simulink model "LQ_integrator_kalman_pendulum_anim"  (Simulink 8.8)
settings: Solver=ode45  StartTime=0.0  StopTime=inf  RelTol=1e-3  EnableMultiTasking=on
values from neighbouring files (symbols this model uses):
  A_kalman = A - L*C    [pendulum_sys_init_solution.m]
  B_kalman = [L B-L*D]    [pendulum_sys_init_solution.m]
  C_kalman = eye(4)    [pendulum_sys_init_solution.m]
  D_kalman = zeros(4,3)    [pendulum_sys_init_solution.m]
  g = 9.81    [pendulum_sys_init_solution.m]
  K_LQ = lqr(A_int,B_int,Q,R)    [pendulum_sys_init_solution.m]
  kc = 2    [pendulum_sys_init_solution.m]
  ke = 2    [pendulum_sys_init_solution.m]
  l = 1    [pendulum_sys_init_solution.m]
  M = 10    [pendulum_sys_init_solution.m]
  m = 2    [pendulum_sys_init_solution.m]
  ra = 10    [pendulum_sys_init_solution.m]
  rr = .1    (= 0.1)    [pendulum_sys_init_solution.m]
undefined symbols (not defined in the file or in its folder): pendolo_sys_diff
libraries: simulink x1, vrlib x1
settings Model: Creator=Titano  LastModifiedBy=AlessioLaBella
settings OptimizationCC: ExpressionDepthLimit=2147483647  InitFltsAndDblsToZero=on
settings DebuggingCC: SolverPrmCheckMsg=warning
settings SimMechanicsCC: VisDuringSimulation=on
settings ConfigurationSet: Description=SimMechanics 2G

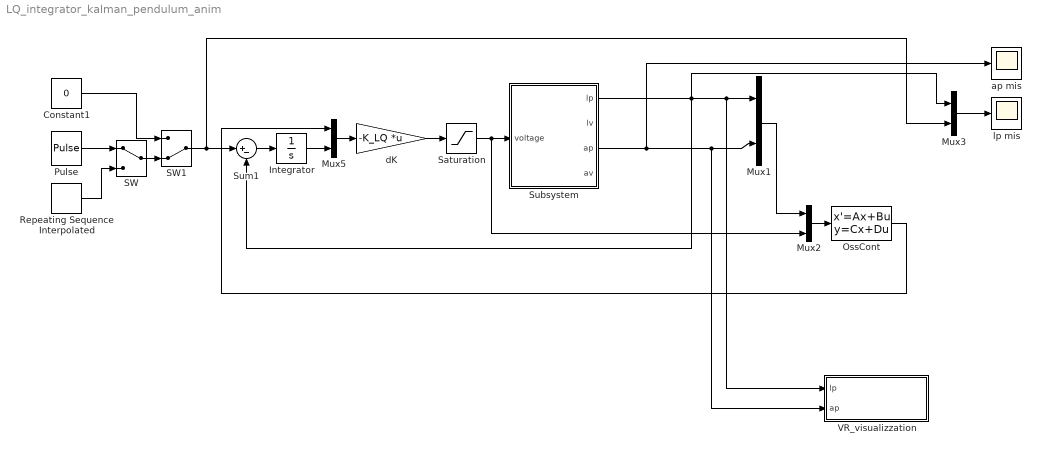
== system LQ_integrator_kalman_pendulum_anim ==
  Constant1 : Constant  Value=0
  Integrator : Integrator
  Mux{1..3,5} (4 alike) : Mux  Inputs=2
  OssCont : StateSpace  A=A_kalman  B=B_kalman  C=C_kalman  D=D_kalman  X0=0
  Pulse : DiscretePulseGenerator  PulseType=Time based  Amplitude=.5  Period=20  PulseWidth=50
  Repeating Sequence Interpolated : simulink/Sources/Repeating Sequence Interpolated  OutValues=[.5 -.5 -.5 .5 .5].'  TimeValues=[0 2.5 5 7.5 10].'  LookUpMeth=Interpolation-Use End Values  tsamp=0.01  OutMin=[]  OutMax=[]  OutDataTypeStr=float('double')  OutputDataTypeScalingMode=Specify via dialog  OutDataType=float('double')  OutScaling=2^-10
  SW : ManualSwitch
  SW1 : ManualSwitch  CurrentSetting=0
  Saturation : Saturate  UpperLimit=24  LowerLimit=-24
  Subsystem : Subsystem
  Sum1 : Sum  Inputs=|+-
  VR_visualizzation : Subsystem
  ap mis : Scope
  dK : Gain  Gain=-K_LQ  Multiplication=Matrix(K*u)
  lp mis : Scope
  wires:
  Mux2/1 -> OssCont/1
  Subsystem/3(ap) -> ap mis/1, Mux1/2, VR_visualizzation/2(ap)
  Subsystem/1(lp) -> Mux3/1, Sum1/2, Mux1/1, VR_visualizzation/1(lp)
  Mux3/1 -> lp mis/1
  Constant1/1 -> SW1/1
  OssCont/1 -> Mux5/1
  SW1/1 -> Mux3/2, Sum1/1
  Sum1/1 -> Integrator/1
  Integrator/1 -> Mux5/2
  dK/1 -> Saturation/1
  Mux5/1 -> dK/1
  Saturation/1 -> Mux2/2, Subsystem/1(voltage)
  SW/1 -> SW1/2
  Pulse/1 -> SW/1
  Repeating Sequence Interpolated/1 -> SW/2
  Mux1/1 -> Mux2/1

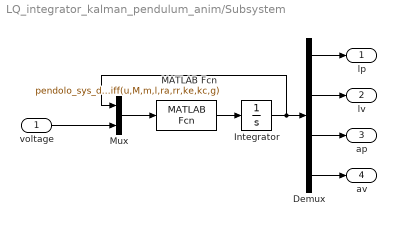
== system LQ_integrator_kalman_pendulum_anim/Subsystem ==
  voltage : Inport
  Demux : Demux
  Integrator : Integrator  InitialCondition=[0 0 0 0]
  MATLAB Fcn : MATLABFcn  MATLABFcn=pendolo_sys_diff(u,M,m,l,ra,rr,ke,kc,g)
  Mux : Mux  Inputs=2
  lp : Outport
  lv : Outport  Port=2
  ap : Outport  Port=3
  av : Outport  Port=4
  wires:
  MATLAB Fcn/1 -> Integrator/1
  Integrator/1 -> Demux/1, Mux/1
  Demux/4 -> av/1
  Demux/3 -> ap/1
  Demux/2 -> lv/1
  Demux/1 -> lp/1
  Mux/1 -> MATLAB Fcn/1
  voltage/1 -> Mux/2

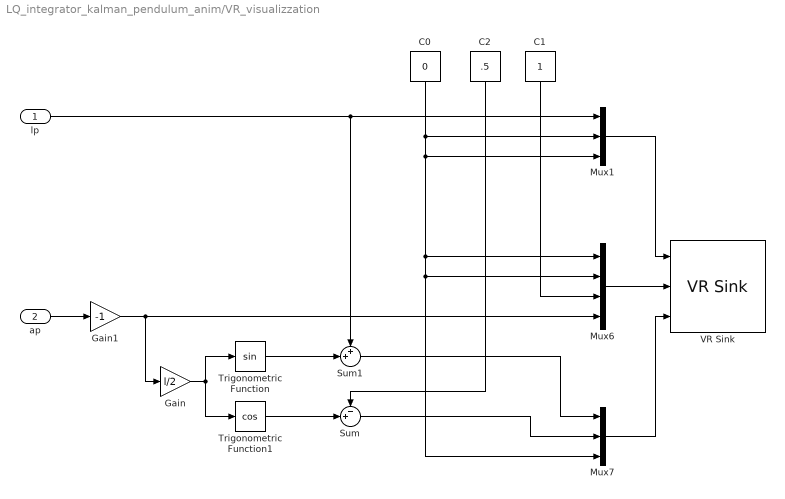
== system LQ_integrator_kalman_pendulum_anim/VR_visualizzation ==
  lp : Inport
  ap : Inport  Port=2
  C0 : Constant  Value=0
  C1 : Constant
  C2 : Constant  Value=.5
  Gain : Gain  Gain=l/2
  Gain1 : Gain  Gain=-1
  Mux1 : Mux  Inputs=3
  Mux6 : Mux
  Mux7 : Mux  Inputs=3
  Sum : Sum  Inputs=-+|
  Sum1 : Sum  Inputs=++|
  Trigonometric Function : Trigonometry
  Trigonometric Function1 : Trigonometry  Operator=cos
  VR Sink : vrlib/VR Sink  InstantiateOnLoad=on  SampleTime=0.02  ViewEnable=on  RemoteChange=off  RemoteView=off  FieldsWritten=carrello.translation.3.1.double#asta.rotation.4.1.double#asta.translation.3.1.double  WorldFileName=vrml1.wrl  AutoView=on  VideoDimensions=[]  AllowVariableSize=off
  wires:
  Mux1/1 -> VR Sink/1
  Mux6/1 -> VR Sink/2
  Mux7/1 -> VR Sink/3
  lp/1 -> Mux1/1, Sum1/1
  C0/1 -> Mux1/2, Mux1/3, Mux6/1, Mux6/2, Mux7/3
  ap/1 -> Gain1/1
  C1/1 -> Mux6/3
  Trigonometric Function/1 -> Sum1/2
  Trigonometric Function1/1 -> Sum/2
  Sum1/1 -> Mux7/1
  Sum/1 -> Mux7/2
  C2/1 -> Sum/1
  Gain/1 -> Trigonometric Function/1, Trigonometric Function1/1
  Gain1/1 -> Mux6/4, Gain/1
